simulink model "HB_Voltage_Feedback"  (R2020a)
settings: Solver=VariableStepAuto  StartTime=0.0  StopTime=1  RelTol=1e-3
undefined symbols (not defined in the file): sigbuilder_block
libraries: powerlib x15, powerlib_meascontrol x1
settings Model: Creator=rajgo  LastModifiedBy=rajgo

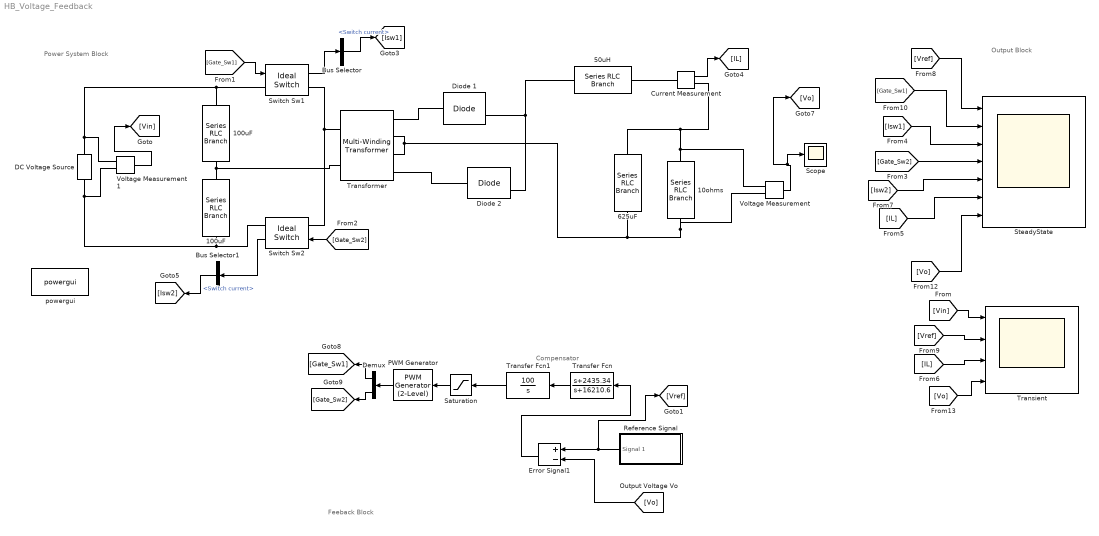
== system HB_Voltage_Feedback ==
  note: Compensator
  note: Output Block
  note: Feeback Block
  note: Power System Block
  100uF : powerlib/Elements/Series RLC Branch  LConnTagsString=__new0  RConnTagsString=__new0  BranchType=RC  Resistance=1e-9  Inductance=1e-3  SetiL0=off  InitialCurrent=0  Capacitance=100e-6  Setx0=off  InitialVoltage=0  Measurements=None
  "100uF " : powerlib/Elements/Series RLC Branch  LConnTagsString=__new0  RConnTagsString=__new0  BranchType=RC  Resistance=1e-9  Inductance=1e-3  SetiL0=off  InitialCurrent=0  Capacitance=100e-6  Setx0=off  InitialVoltage=0  Measurements=None
  10ohms : powerlib/Elements/Series RLC Branch  LConnTagsString=__new0  RConnTagsString=__new0  BranchType=R  Resistance=10  Inductance=1e-3  SetiL0=off  InitialCurrent=0  Capacitance=1e-6  Setx0=off  InitialVoltage=0  Measurements=None
  50uH : powerlib/Elements/Series RLC Branch  LConnTagsString=__new0  RConnTagsString=__new0  BranchType=L  Resistance=1  Inductance=50e-6  SetiL0=off  InitialCurrent=0  Capacitance=1e-6  Setx0=off  InitialVoltage=0  Measurements=None
  625uF : powerlib/Elements/Series RLC Branch  LConnTagsString=__new0  RConnTagsString=__new0  BranchType=C  Resistance=1e-6  Inductance=1e-3  SetiL0=off  InitialCurrent=0  Capacitance=625e-6  Setx0=off  InitialVoltage=18  Measurements=None
  Bus Selector : BusSelector  OutputSignals=Switch current
  Bus Selector1 : BusSelector  OutputSignals=Switch current
  Current Measurement : powerlib/Measurements/Current Measurement  PhasorSimulation=off  OutputType=Complex  PSBequivalent=0
  DC Voltage Source : powerlib/Electrical Sources/DC Voltage Source  Amplitude=40  Measurements=None
  Demux : Demux  Outputs=2
  Diode 1 : powerlib/Power Electronics/Diode  Ron=0.001  Lon=0  Vf=0  IC=0  UseSnubber=0  Rs=500  Cs=250e-9  Measurements=on
  Diode 2 : powerlib/Power Electronics/Diode  Ron=0.001  Lon=0  Vf=0  IC=0  UseSnubber=0  Rs=500  Cs=250e-9  Measurements=on
  Error Signal1 : Sum  Inputs=+-
  PWM Generator : powerlib_meascontrol/Pulse & Signal Generators/PWM Generator (2-Level)  ModulatorType=Single-phase half-bridge (2 pulses)  ModulatorMode=Unsynchronized  Fc=100e3  Pc=90  nF=27  MinMax="[ -1  1 ]"  SamplingTechnique=Natural  ModulatingSignals=off  m=0.8  Freq=60  Phase=0  Ts=0  ShowCarrierOutport=off
  Reference Signal : Subsystem  Tag=STV Subsys  LoadFcn=sigbuilder_block('load');  StartFcn=sigbuilder_block('start');  StopFcn=sigbuilder_block('stop');  ClipboardFcn=sigbuilder_block('clipboard');  mask(Sigbuilder block){tuvar=[0:10]}
      mask help: Simulink:masks:SigbuilderBlock_MD
      mask init:
      | if ~strcmp(get_param(bdroot(gcbh),'SimulationStatus'),'stopped') tuvar = sigbuilder_block('maskInit'); end
      settings: CopyFcn=sigbuilder_block('copy');  DeleteFcn=sigbuilder_block('delete');  ModelCloseFcn=sigbuilder_block('modelClose');  PreSaveFcn=sigbuilder_block('preSave');  PauseFcn=sigbuilder_block('pause');  ContinueFcn=sigbuilder_block('continue');  NameChangeFcn=sigbuilder_block('namechange');  OpenFcn=sigbuilder_block('open',[419.4 157.8 550.8 400.2 ]);  CloseFcn=sigbuilder_block('close');
      mask Display: plot(0, 0, 100, 100,[2, 2, 32, 32, 2], [68, 8, 8, 68, 68],[32, 2], [38, 38], [32, 19, 2],[53, 60, 44], [32, 17, 17, 2],[16, 16, 31, 31]);txt = getActiveGroup(gcbh);text(2, 100, txt,'verticalAlignment', 'top');
  "Saturation " : Saturate  UpperLimit=1  LowerLimit=-1
  Scope : Scope
  SteadyState : Scope  NumInputPorts=7
  Switch Sw1 : powerlib/Power Electronics/Ideal Switch  Ron=0.001  Lon=0  IC=0  Rs=1e5  Cs=inf  Measurements=on
  Switch Sw2 : powerlib/Power Electronics/Ideal Switch  Ron=0.001  Lon=0  IC=0  Rs=1e5  Cs=inf  Measurements=on
  Transfer Fcn : TransferFcn  Numerator=[1 2435.34]  Denominator=[1 16210.6]
  Transfer Fcn1 : TransferFcn  Numerator=[100]  Denominator=[1 0]
  Transformer : powerlib/Elements/Multi-Winding Transformer  LeftWindings=1  RightWindings=2  TappedWindings=no taps  NumberOfTaps=2  SetSaturation=off  Hysteresis=off  DataFile='hysteresis.mat'  Measurements=None  UNITS=SI  NominalPower=[0 0]  NominalVoltages=[ 40 40 40 40 ]  WindingResistances=[0 0 0]  WindingInductances=[0 0 0]  Rm=Inf  Lm=50e-6  Saturation=[0 NaN;0 Inf;0 Inf]  BreakLoop=off  DiscreteSolver=Trapezoidal iterative  DataType=on  InitialFlux=0  TransfoNumber=1
      settings: SourceProductBaseCode=PS
  Transient : Scope  NumInputPorts=4
  Voltage Measurement : powerlib/Measurements/Voltage Measurement  PhasorSimulation=off  OutputType=Complex  PSBequivalent=0
  Voltage Measurement1 : powerlib/Measurements/Voltage Measurement  PhasorSimulation=off  OutputType=Complex  PSBequivalent=0
  powergui : powerlib/powergui  Priority=1  SimulationMode=Continuous  SampleTime=50e-6  frequency=60  Iterations=50  frequencyindice=0  Pbase=100e6  ErrMax=1e-4  UnitsV=kV  UnitsW=MW  buscounter=0  FunctionMessages=off  echomessages=off  EnableUseOfTLC=off  CurrentSourceSwitches=off  DisableSnubberDevices=off  DisableRonSwitches=off  DisableVfSwitches=off  DisplayEquations=off  AutomaticDiscreteSolvers=off  SolverType=Tustin/Backward Euler (TBE)  Interpol=off  ExternalGateDelay=off  methode=off  Ts=100  x0status=blocks  SPID=on  SwTol=0  HookPort=off  NonlinearTolerance=1e-4  nMaxIteration=100  ContinueOnMaxIteration=off  RestoreLinks=warning  ResistiveCurrentMeasurement=off  Frange=[0:2:500]  Ylog=off  Xlog=on  ShowGrid=off  save=off  variable=ZData  structure=0  ZoomFFT=off  StartTime=0.0  cycles=1  DisplayStyle=1  fundamental=60  FreqAxis=off  MaxFrequency=1000  frequencyindicesteady=1  RmsSteady=1  display=off
  wires:
  Voltage Measurement/1 -> [Vo], Scope/1
  Voltage Measurement1/1 -> [Vin]
  Switch Sw1/1 -> Bus Selector/1
  Switch Sw2/1 -> Bus Selector1/1
  Bus Selector1/1 -> [Isw2]  "<Switch current>"
  Current Measurement/1 -> [IL]
  [Vin] -> Transient/1
  [Gate_Sw1] -> Switch Sw1/1
  [Gate_Sw2] -> SteadyState/4
  [Gate_Sw2] -> Switch Sw2/1
  [Isw1] -> SteadyState/3
  Bus Selector/1 -> [Isw1]  "<Switch current>"
  [IL] -> SteadyState/6
  [IL] -> Transient/3
  [Isw2] -> SteadyState/5
  [Vref] -> SteadyState/1
  [Gate_Sw1] -> SteadyState/2
  [Vo] -> SteadyState/7
  [Vo] -> Transient/4
  [Vref] -> Transient/2
  Transfer Fcn/1 -> Transfer Fcn1/1
  Transfer Fcn1/1 -> "Saturation "/1
  "Saturation "/1 -> PWM Generator/1
  PWM Generator/1 -> Demux/1
  Demux/1 -> [Gate_Sw1]
  Demux/2 -> [Gate_Sw2]
  Reference Signal/1(Signal 1) -> [Vref], Error Signal1/1
  [Vo] -> Error Signal1/2
  Error Signal1/1 -> Transfer Fcn/1
  connections:
  "100uF "/LConn1 -- Transformer/LConn2 -- 100uF/RConn1
  100uF/LConn1 -- DC Voltage Source/RConn1 -- Voltage Measurement1/LConn1 -- Switch Sw1/LConn1
  DC Voltage Source/LConn1 -- Switch Sw2/RConn1 -- "100uF "/RConn1 -- Voltage Measurement1/LConn2
  Switch Sw1/RConn1 -- Switch Sw2/LConn1 -- Transformer/LConn1
  Transformer/RConn1 -- Diode 1/LConn1
  Transformer/RConn4 -- Diode 2/LConn1
  Transformer/RConn3 -- 10ohms/RConn1 -- Voltage Measurement/LConn2 -- 625uF/RConn1 -- Transformer/RConn2
  Diode 1/RConn1 -- 50uH/RConn1 -- Diode 2/RConn1
  Voltage Measurement/LConn1 -- 625uF/LConn1 -- Current Measurement/RConn1 -- 10ohms/LConn1
  Current Measurement/LConn1 -- 50uH/LConn1

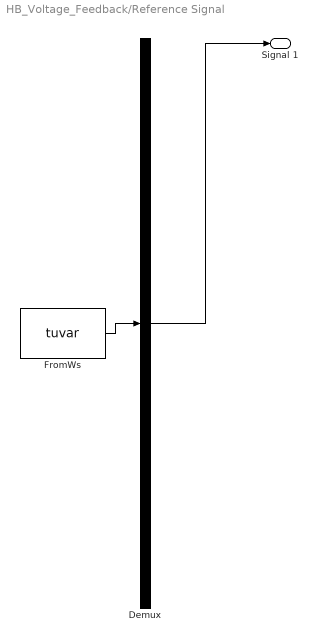
== system HB_Voltage_Feedback/Reference Signal ==
  Demux : Demux  Tag=STV Demux  Outputs=1
      settings: DisplayOption=none
  FromWs : FromWorkspace  Tag=STV FromWs  VariableName=tuvar
      SigBuilderData=|
      | common.afterFinalStr = 'Extrapolate'
      | common.sampleTime = 0
      | dataSet.timeRange = [0 1]
      | dataSet.name = 'Group 1'
      | sbobj.Groups.Name = 'Group 1'
      | sbobj.Groups.Signals.Name = 'Signal 1'
      | sbobj.Groups.Signals.XData = [0 0.5 0.5 1]
      | sbobj.Groups.Signals.YData = [18 18 16 16]
      | sbobj.Groups.TimeRange = [0 1]
  Signal 1 : Outport  Tag=STV Outport
  wires:
  Demux/1 -> Signal 1/1
  FromWs/1 -> Demux/1
